simulink model "Teil_b"  (R2014b)
settings: Solver=VariableStepAuto  StartTime=0.0  StopTime=10.0  RelTol=1e-3
settings Model: Creator=sephkleg  LastModifiedBy=cweber
settings DataIOCC: LimitDataPoints=off  SaveFormat=Dataset
settings OptimizationCC: UseDivisionForNetSlopeComputation=off  LifeSpan=auto  SimCompilerOptimization=off
settings DebuggingCC: SolverPrmCheckMsg=none  FcnCallInpInsideContextMsg=error  FrameProcessingCompatibilityMsg=error  SFUnexpectedBacktrackingDiag=error  SFNoUnconditionalDefaultTransitionDiag=error
settings HardwareCC: ProdBitPerPointer=64  ProdLargestAtomicFloat=Float  ProdIntDivRoundTo=Zero  ProdEndianess=LittleEndian  ProdWordSize=64  ProdHWDeviceType=Intel->x86-64 (Windows64)
settings ModelReferenceCC: PropagateSignalLabelsOutOfModel=on
settings RTWCC: RTWCompilerOptimization=off
settings GRTTargetCC: TargetLangStandard=C99 (ISO)  GeneratePreprocessorConditionals=Use local settings

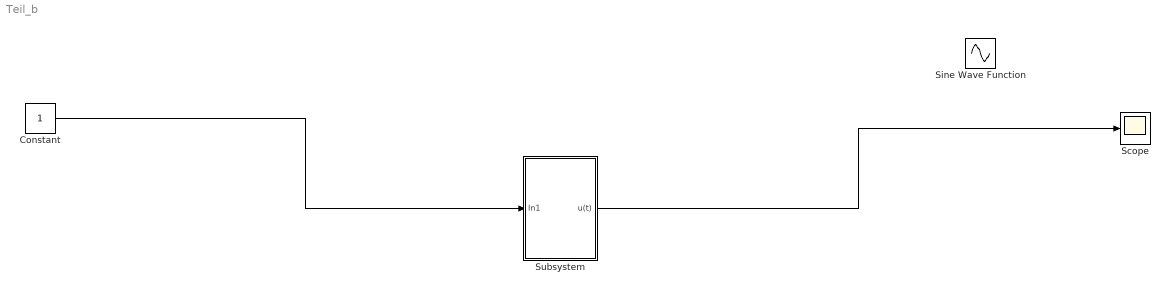
== system Teil_b ==
  Constant : Constant
  Scope : Scope
      settings: YMin=-10  YMax=10
  Sine Wave Function : Sin  TimeSource=Use external signal  SampleTime=0
  Subsystem : Subsystem
  wires:
  Constant/1 -> Subsystem/1(In1)
  Subsystem/1(u(t)) -> Scope/1

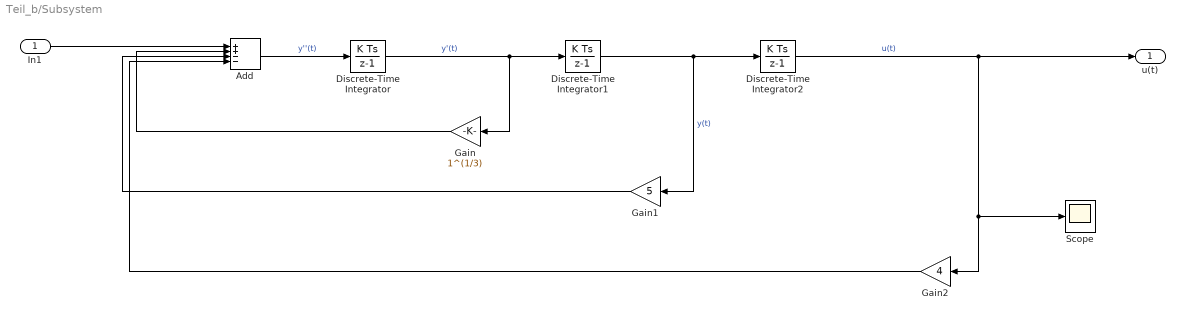
== system Teil_b/Subsystem ==
  In1 : Inport
  Add : Sum  Inputs=++--
  Discrete-Time Integrator : DiscreteIntegrator  InitialConditionSetting=State (most efficient)  SampleTime=-1
  Discrete-Time Integrator1 : DiscreteIntegrator  InitialConditionSetting=State (most efficient)  SampleTime=-1
  Discrete-Time Integrator2 : DiscreteIntegrator  InitialConditionSetting=State (most efficient)  SampleTime=-1
  Gain : Gain  Gain=1^(1/3)
  Gain1 : Gain  Gain=5
  Gain2 : Gain  Gain=4
  Scope : Scope
  u(t) : Outport
  wires:
  Discrete-Time Integrator2/1 -> u(t)/1, Scope/1, Gain2/1  "u(t)"
  Gain2/1 -> Add/4
  Discrete-Time Integrator/1 -> Gain/1, Discrete-Time Integrator1/1  "y'(t)"
  In1/1 -> Add/1
  Gain1/1 -> Add/3
  Gain/1 -> Add/2
  Add/1 -> Discrete-Time Integrator/1  "y''(t)"
  Discrete-Time Integrator1/1 -> Gain1/1, Discrete-Time Integrator2/1  "y(t)"
